simulink model "Multi_Level_H_Bridge_3"  (R2014a)
settings: Solver=ode45  StartTime=0.0  StopTime=0.06  RelTol=1e-3
libraries: powerlib x9
settings Model: Creator=RAVINDERNATH YADAV  LastModifiedBy=RAVINDERNATH YADAV

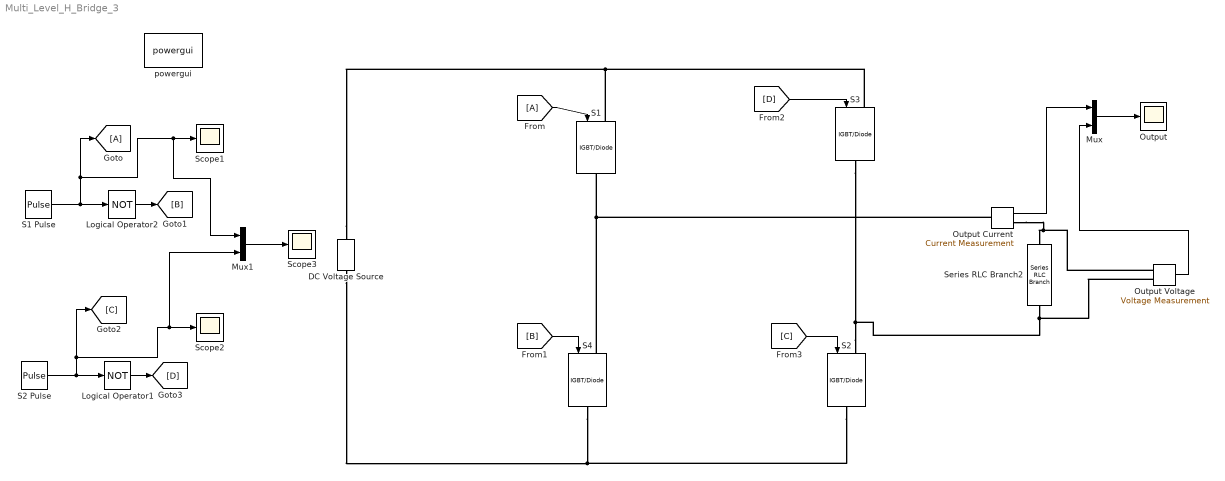
== system Multi_Level_H_Bridge_3 ==
  DC Voltage Source : powerlib/Electrical Sources/DC Voltage Source  Amplitude=2  Measurements=None
  Logical Operator1 : Logic  Operator=NOT  AllPortsSameDT=off  OutDataTypeStr=boolean
  Logical Operator2 : Logic  Operator=NOT  AllPortsSameDT=off  OutDataTypeStr=boolean
  Mux : Mux  Inputs=2
  Mux1 : Mux  Inputs=2
  Output : Scope
      settings: ShowLegends=on  YMin=-200  YMax=200
  Output Current : powerlib/Measurements/Current Measurement  PhasorSimulation=off  OutputType=Complex  PSBequivalent=0
  Output Voltage : powerlib/Measurements/Voltage Measurement  PhasorSimulation=off  OutputType=Complex  PSBequivalent=0
  S{1..4} (4 alike) : powerlib/Power Electronics/IGBT//Diode  Ron=1e-3  Rs=1e5  Cs=inf  Measurements=off
  "S1 Pulse " : DiscretePulseGenerator  PulseType=Time based  Period=0.01  PulseWidth=50
  "S2 Pulse " : DiscretePulseGenerator  PulseType=Time based  Period=0.01  PulseWidth=50  PhaseDelay=0.0025
  Scope1 : Scope
      settings: YMin=-200  YMax=200
  Scope2 : Scope
      settings: YMin=-200  YMax=200  SaveName=ScopeData2
  Scope3 : Scope
      settings: ShowLegends=on  YMin=-0.5  YMax=1.5  SaveName=ScopeData3
  Series RLC Branch2 : powerlib/Elements/Series RLC Branch  LConnTagsString=__new0  RConnTagsString=__new0  BranchType=R  Resistance=10  Inductance=1e-3  SetiL0=off  InitialCurrent=0  Capacitance=1e-6  Setx0=off  InitialVoltage=0  Measurements=None
  powergui : powerlib/powergui  Priority=1  SimulationMode=Discrete  SolverType=Tustin  SampleTime=50e-6  frequency=60  SPID=off  DisableSnubberDevices=off  DisableRonSwitches=off  DisableVfSwitches=off  SwTol=0  Interpol=off  DisplayEquations=off  Ts=0  methode=off  frequencyindice=0  Pbase=100e6  ErrMax=1e-4  Iterations=50  UnitsV=kV  UnitsW=MW  FunctionMessages=off  echomessages=off  HookPort=off  EnableUseOfTLC=off  x0status=blocks  RestoreLinks=warning  ResistiveCurrentMeasurement=off  Frange=[0:2:500]  Ylog=off  Xlog=on  ShowGrid=off  save=off  variable=ZData  structure=0  ZoomFFT=off  StartTime=0.0  cycles=1  DisplayStyle=1  fundamental=60  FreqAxis=off  MaxFrequency=1000  frequencyindicesteady=1  RmsSteady=1  display=off
  wires:
  Mux/1 -> Output/1
  Output Voltage/1 -> Mux/2
  Output Current/1 -> Mux/1
  "S1 Pulse "/1 -> Mux1/1, Scope1/1, [A], Logical Operator2/1
  Logical Operator2/1 -> [B]
  [A] -> S1/1
  [B] -> S4/1
  "S2 Pulse "/1 -> Mux1/2, Scope2/1, [C], Logical Operator1/1
  Logical Operator1/1 -> [D]
  [D] -> S3/1
  [C] -> S2/1
  Mux1/1 -> Scope3/1
  connections:
  DC Voltage Source/LConn1 -- S2/RConn1 -- S4/RConn1
  S4/LConn1 -- Output Current/LConn1 -- S1/RConn1
  DC Voltage Source/RConn1 -- S3/LConn1 -- S1/LConn1
  S2/LConn1 -- Output Voltage/LConn2 -- Series RLC Branch2/RConn1 -- S3/RConn1
  Output Voltage/LConn1 -- Output Current/RConn1 -- Series RLC Branch2/LConn1
